simulink model "NumberPlateV2"  (R2022a)
settings: Solver=VariableStepAuto  StartTime=0.0  StopTime=10.0  RelTol=1e-3
undefined symbols (not defined in the file): sigbuilder_block
libraries: simulink x6
settings Model: Creator=riya4  LastModifiedBy=riya4

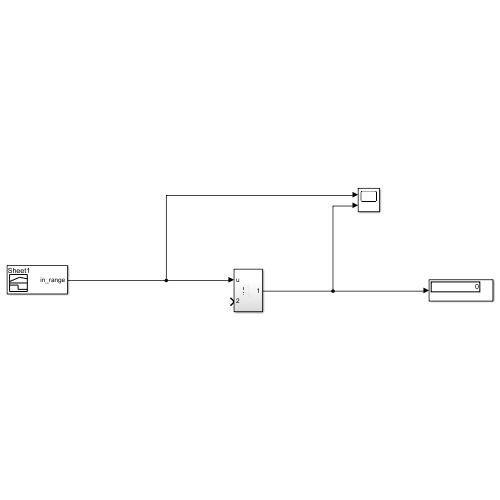
[thumbnail: Simulink's stored preview of the top-level diagram]
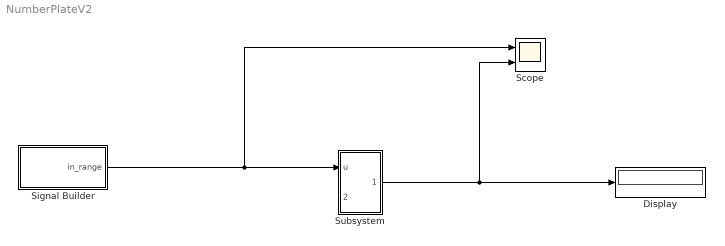
== system NumberPlateV2 ==
  Display : Display
  Scope : Scope  NumInputPorts=2
  Signal Builder : Subsystem  Tag=STV Subsys  LoadFcn=sigbuilder_block('load',[437.6 199.2 550.4 400 ]);  StartFcn=sigbuilder_block('start');  StopFcn=sigbuilder_block('stop');  ClipboardFcn=sigbuilder_block('clipboard');  mask(Sigbuilder block){tuvar=[0:10]}
      mask help: Simulink:masks:SigbuilderBlock_MD
      mask init:
      | if ~strcmp(get_param(bdroot(gcbh),'SimulationStatus'),'stopped') tuvar = sigbuilder_block('maskInit'); end
      settings: CopyFcn=sigbuilder_block('copy');  DeleteFcn=sigbuilder_block('delete');  ModelCloseFcn=sigbuilder_block('modelClose');  PreSaveFcn=sigbuilder_block('preSave');  PauseFcn=sigbuilder_block('pause');  ContinueFcn=sigbuilder_block('continue');  NameChangeFcn=sigbuilder_block('namechange');  OpenFcn=sigbuilder_block('open',[437.6 199.2 550.4 400 ]);  CloseFcn=sigbuilder_block('close');
      mask Display: plot(0, 0, 100, 100,[2, 2, 32, 32, 2], [68, 8, 8, 68, 68],[32, 2], [38, 38], [32, 19, 2],[53, 60, 44], [32, 17, 17, 2],[16, 16, 31, 31]);txt = getActiveGroup(gcbh);text(2, 100, txt,'verticalAlignment', 'top');
  Subsystem : Subsystem
  wires:
  Signal Builder/1(in_range) -> Scope/1, Subsystem/1(u)
  Subsystem/1(Out1) -> Scope/2, Display/1

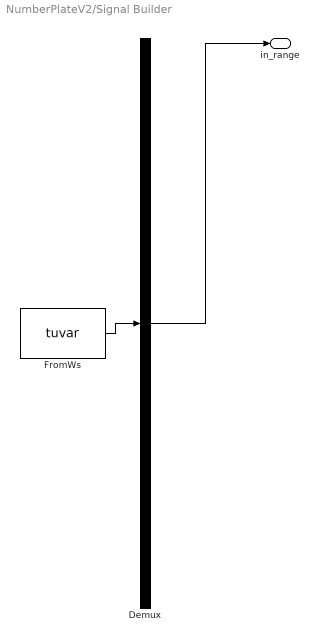
== system NumberPlateV2/Signal Builder ==
  Demux : Demux  Tag=STV Demux  Outputs=1
      settings: DisplayOption=none
  FromWs : FromWorkspace  Tag=STV FromWs  VariableName=tuvar
      SigBuilderData=|
      | common.afterFinalStr = 'Extrapolate'
      | common.sampleTime = 0
      | dataSet.timeRange = [1 9]
      | dataSet.name = 'Sheet1'
      | sbobj.Groups.Name = 'Sheet1'
      | sbobj.Groups.Signals.Name = 'in_range'
      | sbobj.Groups.Signals.XData = [1 2 3 4 5 6 7 8 9]
      | sbobj.Groups.Signals.YData = [0 1 1 0 0 1 1 0 0]
  in_range : Outport  Tag=STV Outport
  wires:
  Demux/1 -> in_range/1
  FromWs/1 -> Demux/1

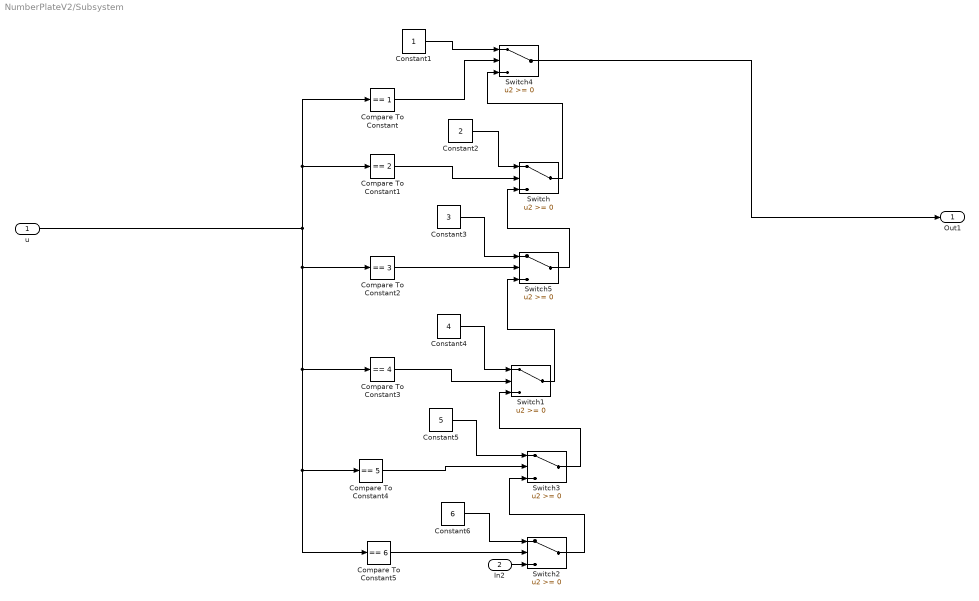
== system NumberPlateV2/Subsystem ==
  u : Inport
  In2 : Inport  Port=2
  Compare To Constant : simulink/Logic and Bit Operations/Compare To Constant  relop===  const=1  OutDataTypeStr=boolean
  Compare To Constant1 : simulink/Logic and Bit Operations/Compare To Constant  relop===  const=2  OutDataTypeStr=boolean
  Compare To Constant2 : simulink/Logic and Bit Operations/Compare To Constant  relop===  const=3  OutDataTypeStr=boolean
  Compare To Constant3 : simulink/Logic and Bit Operations/Compare To Constant  relop===  const=4  OutDataTypeStr=boolean
  Compare To Constant4 : simulink/Logic and Bit Operations/Compare To Constant  relop===  const=5  OutDataTypeStr=boolean
  Compare To Constant5 : simulink/Logic and Bit Operations/Compare To Constant  relop===  const=6  OutDataTypeStr=boolean
  Constant1 : Constant
  Constant2 : Constant  Value=2
  Constant3 : Constant  Value=3
  Constant4 : Constant  Value=4
  Constant5 : Constant  Value=5
  Constant6 : Constant  Value=6
  Switch{,1..5} (6 alike) : Switch  SaturateOnIntegerOverflow=off  InputSameDT=off
  Out1 : Outport
  wires:
  Compare To Constant3/1 -> Switch1/2
  Compare To Constant/1 -> Switch4/2
  Switch1/1 -> Switch5/3
  Compare To Constant2/1 -> Switch5/2
  Switch2/1 -> Switch3/3
  u/1 -> Compare To Constant5/1, Compare To Constant4/1, Compare To Constant3/1, Compare To Constant2/1, Compare To Constant/1, Compare To Constant1/1
  Switch4/1 -> Out1/1
  Compare To Constant4/1 -> Switch3/2
  Compare To Constant5/1 -> Switch2/2
  Compare To Constant1/1 -> Switch/2
  Switch3/1 -> Switch1/3
  Switch5/1 -> Switch/3
  Switch/1 -> Switch4/3
  Constant1/1 -> Switch4/1
  Constant2/1 -> Switch/1
  Constant4/1 -> Switch1/1
  Constant3/1 -> Switch5/1
  Constant5/1 -> Switch3/1
  Constant6/1 -> Switch2/1
  In2/1 -> Switch2/3
